simulink model "power_13NodeTestFeedermodel"  (R2021b)
settings: Solver=ode45  StartTime=0.0  StopTime=16  MaxStep=0.04  RelTol=1e-3
PreLoadFcn:
  | power_13NodeTestFeeder_init;
  | Ts=50e-6
values from neighbouring files (symbols this model uses):
  C_dc = 0.008*(n)    (= 1.6)    [VSM.m]
  C_f = n*300*10^-6    (= 0.06)    [VSM.m]
  D_p = (1/(m_p*w_b))    (= 844.343197019)    [VSM.m]
  i_ll = -1.15*(S_b/Vdc_n)-i_loss_dc    [VSM.m]
  i_ul = 1.15*(S_b/Vdc_n)+i_loss_dc    [VSM.m]
  J = D_p*tau_f    (= 16.8868639404)    [VSM.m]
  k_dc = eta_1/(Vdc_n*m_p)    [VSM.m]
  K_p = (1/Vdc_n)    [VSM.m]
  K_r = 1/R_dc    [VSM.m]
  Kff_i = 1    [VSM.m]
  Kff_v = 1    [VSM.m]
  Ki_i = (1/n)*1.19    (= 0.00595)    [VSM.m]
  Ki_v = (n)*1.161022    (= 232.2044)    [VSM.m]
  ki_v_ac = 4*5.2500e-04    (= 0.0021)    [VSM.m]
  Kp_i = 0.738891    [VSM.m]
  Kp_v = 0.52    [VSM.m]
  kp_v_ac = 0.001    [VSM.m]
  L_f = (1/n)*200*10^-6    (= 1e-06)    [VSM.m]
  n = 200    [VSM.m]
  ps = base/3    (= 0.75)    [VSM.m]
  R_dc = (Vdc_n/(0.05*(S_b)/Vdc_n))    [VSM.m]
  R_f = 0.001/n    (= 5e-06)    [VSM.m]
  S_b = 1*(10^6)    (= 1000000)    [VSM.m]
  T_en = T_load-0.5    (= 24.5)    [VSM.m]
  tau_dc = 0.05    [VSM.m]
  V_m = sqrt(2/3)*V1_rms    [VSM.m]
  Vdc_n = 3*V_m    [VSM.m]
  w_b = 2*pi*f_b    (= 376.991118431)    [VSM.m]
  w_f = 2*pi*60    (= 376.991118431)    [VSM.m]
undefined symbols (not defined in the file or in its folder): C_601, C_602, C_603, C_604, C_605, C_606, C_607, ft2km, i_dc, L_601, L_602, L_603, L_604, L_605, L_606, L_607, R_601, R_602, R_603, R_604, R_605, R_606, R_607
libraries: spsSeriesRLCBranchLib x16, spsabctodq0Lib x16, spsVoltageMeasurementLib x14, spsCurrentMeasurementLib x12, spsGroundLib x12, spsLoadFlowBusLib x12, spsPiSectionLineLib x9, spsThreePhaseSeriesRLCLoadLib x7, spsMultimeterLib x6, spsPowerPhasorLib x6, spsThreePhaseVIMeasurementLib x5, spsSeriesRLCLoadLib x5
(part 1 of 2)
settings Model: Creator=The MathWorks, Inc.  LastModifiedBy=aes21009
settings SolverCC: ZeroCrossAlgorithm=Adaptive  AlgebraicLoopSolver=TrustRegion
settings DataIOCC: ExternalInput=getinputstruct(op_IEEE_13_node_5)  InitialState=getstatestruct(op_IEEE_13_node_5)  LimitDataPoints=on  SaveFormat=Array  ReturnWorkspaceOutputs=off
settings OptimizationCC: LifeSpan=inf
settings DebuggingCC: AlgebraicLoopMsg=none  IgnoredZcDiagnostic=none  FcnCallInpInsideContextMsg=warning  UnconnectedInputMsg=none  UnconnectedOutputMsg=none  UnconnectedLineMsg=none  StateNameClashWarn=warning  SFUnexpectedBacktrackingDiag=warning  SFNoUnconditionalDefaultTransitionDiag=warning  SFExecutionAtInitializationDiag=none  SFMachineParentedDataDiag=warning
settings ModelReferenceCC: PropagateSignalLabelsOutOfModel=off
settings SFSimCC: CustomCodeUndefinedFunction=UseInterfaceOnly
settings CodeAppCC: StateflowObjectComments=on
settings SimscapeCC: SimscapeNormalizeSystem=off

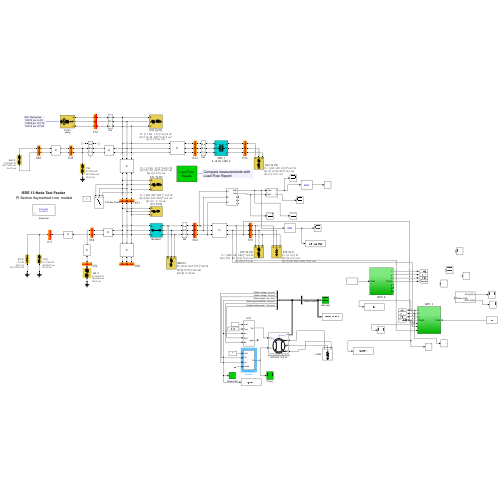
[thumbnail: Simulink's stored preview of the top-level diagram]
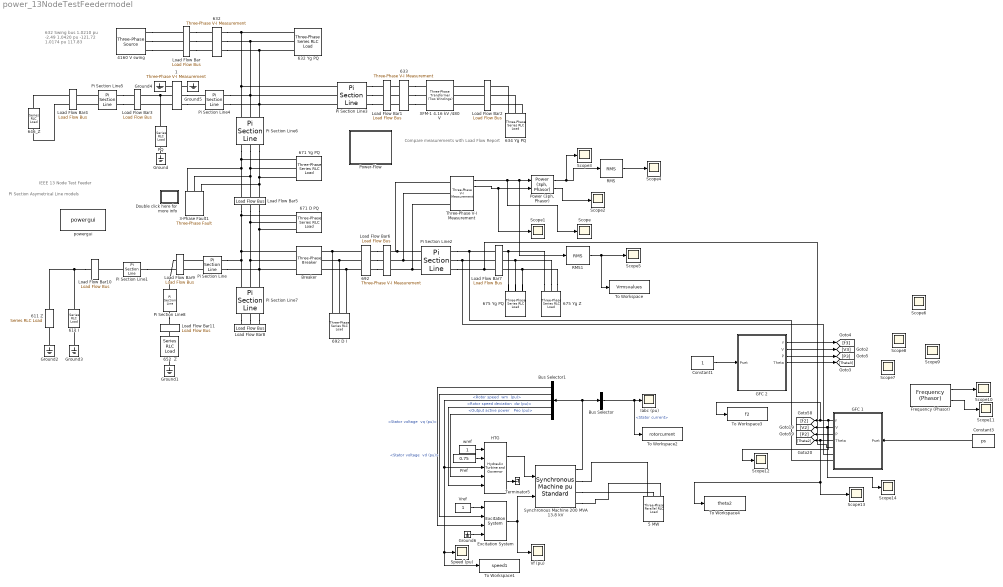
== system power_13NodeTestFeedermodel ==
  note: Compare measurements with
      | Load Flow Report
  note: 632 Swing bus
      | 1.0210 pu -2.49
      | 1.0420 pu -121.72
      | 1.0174 pu 117.83
  note: PI Section Asymetrical Line models
  note: IEEE 13 Node Test Feeder
  " 634 Yg PQ " : spsThreePhaseSeriesRLCLoadLib/Three-Phase Series RLC Load  LConnTagsString=A|B|C  Configuration=Y (grounded)  NominalVoltage=120e3  Vabc=[ 0.993926 1.02168 0.995885]*277.128  Vabcp=[1e3 1e3 1e3]  NominalFrequency=60  UnbalancedPower=on  ActivePower=1e+006  InductivePower=0  CapacitivePower=0  Pabc=[160 120 120]*1e3  QLabc=[110 90 90]*1e3  QCabc=[0 0 0]  Pabcp=[10e3 9e3 11e3]  QLabcp=[100 90 110]  QCabcp=[100 90 110]  Measurements=None  LoadType=constant PQ
      settings: AttributesFormatString=|
      | P= %<Pabc> W
      | Ql=%<QLabc> var
      | Qc=%<QCabc> var
  " Iabc (pu)" : Scope
  " Speed (pu)" : Scope
  1 : spsThreePhaseVIMeasurementLib/Three-Phase V-I Measurement  VoltageMeasurement=phase-to-ground  SetLabelV=on  LabelV=Vabc_645  Vpu=off  VpuLL=off  CurrentMeasurement=yes  SetLabelI=on  LabelI=Iabc_645  Ipu=off  Pbase=100e6  Vbase=4160  OutputType=Complex  PhasorSimulation=off  PSBequivalent=0
  3-Phase Fault1 : spsThreePhaseFaultLib/Three-Phase Fault  InitialStates=0  FaultA=on  FaultB=on  FaultC=on  GroundFault=on  SwitchTimes=[10.1 10.2]  External=off  SwitchStatus=NaN  FaultResistance=1e-3  GroundResistance=1e-3  SnubberResistance=inf  SnubberCapacitance=inf  Measurements=None
  4160 V swing : spsThreePhaseSourceLib/Three-Phase Source  InternalConnection=Yg  VoltagePhases=on  Voltage=120e3  PhaseAngle=0  Voltage_phases=[ 1.021 1.042 1.0174]*2401.78  PhaseAngles_phases=[ -2.49006 -121.72 117.83]  Frequency=60  NonIdealSource=on  SpecifyImpedance=off  Resistance=1e-5  Inductance=0  ShortCircuitLevel=100e6  BaseVoltage=120e3  XRratio=10  BusType=swing  Pref=0  Qref=0  Prefabc=[0 0 0]  Qrefabc=[0 0 0]  Qmin="[-inf  -inf -inf]"  Qmax="[inf  inf inf]"
  5 MW : spsThreePhaseParallelRLCLoadLib/Three-Phase Parallel RLC Load  LConnTagsString=A|B|C  Configuration=Y (grounded)  NominalVoltage=4160  Vabc=[1e3 1e3 1e3]  Vabcp=[1e3 1e3 1e3]  NominalFrequency=60  UnbalancedPower=off  ActivePower=50000  InductivePower=0  CapacitivePower=0  Pabc=[10e3 9e3 11e3]  QLabc=[100 90 110]  QCabc=[100 90 110]  Pabcp=[10e3 9e3 11e3]  QLabcp=[100 90 110]  QCabcp=[100 90 110]  Measurements=None  LoadType=constant Z
  611 I : spsSeriesRLCLoadLib/Series RLC Load  LConnTagsString=a  RConnTagsString=__new0  NominalVoltage=0.986755*2401.78  NominalFrequency=60  ActivePower=170e3  InductivePower=80e3  CapacitivePower=0  Setx0=off  InitialVoltage=0  SetiL0=off  InitialCurrent=0  Measurements=Branch voltage and current  LoadType=constant I
      settings: AttributesFormatString=|
      | P=%<ActivePower> W
      | Ql=%<InductivePower> var
      | Qc=%<CapacitivePower> var
  611 Z : spsSeriesRLCLoadLib/Series RLC Load  LConnTagsString=a  RConnTagsString=__new0  NominalVoltage=4160/sqrt(3)  NominalFrequency=60  ActivePower=0  InductivePower=0  CapacitivePower=100e3  Setx0=off  InitialVoltage=0  SetiL0=off  InitialCurrent=0  Measurements=None  LoadType=constant Z
      settings: AttributesFormatString=|
      | P=%<ActivePower> W
      | Ql=%<InductivePower> var
      | Qc=%<CapacitivePower> var
  632 : spsThreePhaseVIMeasurementLib/Three-Phase V-I Measurement  VoltageMeasurement=phase-to-ground  SetLabelV=on  LabelV=Vabc_632  Vpu=off  VpuLL=off  CurrentMeasurement=yes  SetLabelI=on  LabelI=Iabc_632  Ipu=off  Pbase=100e6  Vbase=4160  OutputType=Complex  PhasorSimulation=off  PSBequivalent=0
  632 Yg PQ : spsThreePhaseSeriesRLCLoadLib/Three-Phase Series RLC Load  LConnTagsString=A|B|C  Configuration=Y (grounded)  NominalVoltage=120e3  Vabc=[ 1.021 1.042 1.0174]*2401.78  Vabcp=[1e3 1e3 1e3]  NominalFrequency=60  UnbalancedPower=on  ActivePower=1e+006  InductivePower=0  CapacitivePower=0  Pabc="[17 66  117]*1e3/2"  QLabc="[10 38  68]*1e3/2"  QCabc=[0 0 0]  Pabcp=[10e3 9e3 11e3]  QLabcp=[100 90 110]  QCabcp=[100 90 110]  Measurements=None  LoadType=constant PQ
      settings: AttributesFormatString=|
      | P= %<Pabc> W
      | Ql=%<QLabc> var
      | Qc=%<QCabc> var
  633 : spsThreePhaseVIMeasurementLib/Three-Phase V-I Measurement  VoltageMeasurement=phase-to-ground  SetLabelV=on  LabelV=Vabc_633  Vpu=off  VpuLL=off  CurrentMeasurement=yes  SetLabelI=on  LabelI=Iabc_633  Ipu=off  Pbase=100e6  Vbase=4160  OutputType=Complex  PhasorSimulation=off  PSBequivalent=0
  646_Z : spsSeriesRLCLoadLib/Series RLC Load  LConnTagsString=a  RConnTagsString=__new0  NominalVoltage=4160  NominalFrequency=60  ActivePower=230e3  InductivePower=132e3  CapacitivePower=0  Setx0=off  InitialVoltage=0  SetiL0=off  InitialCurrent=0  Measurements=None  LoadType=constant Z
      settings: AttributesFormatString=|
      | P=%<ActivePower> W
      | Ql=%<InductivePower> var
      | Qc=%<CapacitivePower> var
  "652  Z " : spsSeriesRLCLoadLib/Series RLC Load  LConnTagsString=a  RConnTagsString=__new0  NominalVoltage=4160/sqrt(3)  NominalFrequency=60  ActivePower=128e3  InductivePower=86e3  CapacitivePower=0  Setx0=off  InitialVoltage=0  SetiL0=off  InitialCurrent=0  Measurements=None  LoadType=constant Z
      settings: AttributesFormatString=|
      | P=%<ActivePower> W
      | Ql=%<InductivePower> var
      | Qc=%<CapacitivePower> var
  671 D PQ : spsThreePhaseSeriesRLCLoadLib/Three-Phase Series RLC Load  LConnTagsString=A|B|C  Configuration=Delta  NominalVoltage=120e3  Vabc="[1  1  1]*120e3/sqrt(3)"  Vabcp=[ 1.7426 1.77325 1.71534]*2401.78  NominalFrequency=60  UnbalancedPower=on  ActivePower=1e+006  InductivePower=0  CapacitivePower=0  Pabc="[17 66  117]*1e3/2"  QLabc="[10 38  68]*1e3/2"  QCabc=[0 0 0]  Pabcp=[385 385 385 ]*1e3  QLabcp=[220 220 220]*1e3  QCabcp="[0  0  0]"  Measurements=Branch voltages and currents  LoadType=constant PQ
      settings: AttributesFormatString=|
      | P= %<Pabcp> W
      | Ql=%<QLabcp> var
      | Qc=%<QCabcp> var
  671 Yg PQ : spsThreePhaseSeriesRLCLoadLib/Three-Phase Series RLC Load  LConnTagsString=A|B|C  Configuration=Y (grounded)  NominalVoltage=120e3  Vabc=[ 0.990007 1.05293 0.977696]*2401.78  Vabcp=[1e3 1e3 1e3]  NominalFrequency=60  UnbalancedPower=on  ActivePower=1e+006  InductivePower=0  CapacitivePower=0  Pabc="[17 66  117]*1e3/2"  QLabc="[10 38  68]*1e3/2"  QCabc=[0 0 0]  Pabcp=[10e3 9e3 11e3]  QLabcp=[100 90 110]  QCabcp=[100 90 110]  Measurements=None  LoadType=constant PQ
      settings: AttributesFormatString=|
      | P= %<Pabc> W
      | Ql=%<QLabc> var
      | Qc=%<QCabc> var
  675 Yg PQ : spsThreePhaseSeriesRLCLoadLib/Three-Phase Series RLC Load  LConnTagsString=A|B|C  Configuration=Y (grounded)  NominalVoltage=120e3  Vabc=[ 0.983621 1.05532 0.975578]*2401.78  Vabcp=[1e3 1e3 1e3]  NominalFrequency=60  UnbalancedPower=on  ActivePower=1e+006  InductivePower=0  CapacitivePower=0  Pabc="[485  68  290]*1e3"  QLabc="[190  60  212]*1e3"  QCabc=[0 0 0]  Pabcp=[10e3 9e3 11e3]  QLabcp=[100 90 110]  QCabcp=[100 90 110]  Measurements=Branch voltages and currents  LoadType=constant PQ
      settings: AttributesFormatString=|
      | P= %<Pabc> W
      | Ql=%<QLabc> var
      | Qc=%<QCabc> var
  675 Yg Z : spsThreePhaseSeriesRLCLoadLib/Three-Phase Series RLC Load  LConnTagsString=A|B|C  Configuration=Y (grounded)  NominalVoltage=120e3  Vabc="[1  1  1]*4160/sqrt(3)"  Vabcp=[1e3 1e3 1e3]  NominalFrequency=60  UnbalancedPower=on  ActivePower=1e+006  InductivePower=0  CapacitivePower=0  Pabc=[0 0 0]  QLabc=[0 0 0]  QCabc=[200 200 200]*1e3  Pabcp=[10e3 9e3 11e3]  QLabcp=[100 90 110]  QCabcp=[100 90 110]  Measurements=None  LoadType=constant Z
      settings: AttributesFormatString=|
      | P= %<Pabc> W
      | Ql=%<QLabc> var
      | Qc=%<QCabc> var
  692 : spsThreePhaseVIMeasurementLib/Three-Phase V-I Measurement  VoltageMeasurement=phase-to-ground  SetLabelV=on  LabelV=Vabc_692  Vpu=off  VpuLL=off  CurrentMeasurement=yes  SetLabelI=on  LabelI=Iabc_692  Ipu=off  Pbase=100e6  Vbase=4160  OutputType=Complex  PhasorSimulation=off  PSBequivalent=0
  692 D I : spsThreePhaseSeriesRLCLoadLib/Three-Phase Series RLC Load  LConnTagsString=A|B|C  Configuration=Delta  NominalVoltage=120e3  Vabc="[1  1  1]*120e3/sqrt(3)"  Vabcp=[ 1.73731 1.75253 1.72367]*2401.78  NominalFrequency=60  UnbalancedPower=on  ActivePower=1e+006  InductivePower=0  CapacitivePower=0  Pabc="[17 66  117]*1e3/2"  QLabc="[10 38  68]*1e3/2"  QCabc=[0 0 0]  Pabcp=[1e-6 1e-6 170 ]*1e3  QLabcp=[0 0 151]*1e3  QCabcp="[0  0  0]"  Measurements=Branch voltages and currents  LoadType=constant I
      settings: AttributesFormatString=|
      | P= %<Pabcp> W
      | Ql=%<QLabcp> var
      | Qc=%<QCabcp> var
  Breaker : spsThreePhaseBreakerLib/Three-Phase Breaker  InitialState=closed  SwitchA=on  SwitchB=on  SwitchC=on  SwitchTimes=[ 12 ]  External=off  BreakerResistance=0.0001  SnubberResistance=inf  SnubberCapacitance=0  Measurements=Breaker voltages and currents
  Bus Selector : BusSelector  OutputSignals=Stator current
  Bus Selector1 : BusSelector  OutputSignals="dq0 components.Stator voltage  vq (pu),dq0 components.Stator voltage  vd (pu),Mechanical.Rotor speed  wm  (pu),Mechanical.Rotor speed deviation  dw (pu),Output active power   Peo (pu)"
  Constant1 : Constant
  Constant3 : Constant  Value=ps
  Double click here for more info : Subsystem
      settings: OpenFcn=showdemo(bdroot(gcb))
      mask Display: disp('?')
  Excitation System : spsExcitationSystemLib/Excitation System  tr=20e-3  reg=[ 300, 0.001 ]  exc=[ 1, 0 ]  tgr=[ 0, 0 ]  damp=[ 0.001, 0.1 ]  sat=[ 0, 0 ]  lim=[ -11.5, 11.5, 0 ]  v0=[1,1.29071]
      settings: SourceProductBaseCode=PS
  Frequency (Phasor) : spsFrequencyPhasorLib/Frequency (Phasor)  Fn=60  T=0.1
      settings: SourceProductBaseCode=PS
  GFC 1 : Subsystem
  GFC 2 : Subsystem
  Ground{,1..5} (6 alike) : spsGroundLib/Ground  LConnTagsString=a
  Ground6 : Ground
  HTG : spsHydraulicTurbineandGovernorLib/Hydraulic Turbine and Governor  sm="[ 10/3  0.07 ]"  gate="[  0.01  0.97518  -0.1  0.1 ]"  reg="[  0.05  1.163  0.105  0  0.01  ]"  hyd="[  0  2.67  ]"  dref=0  po=0.751606
      settings: SourceProductBaseCode=PS
  Load Flow Bar : spsLoadFlowBusLib/Load Flow Bus  LConnTagsString=a|b|c  RConnTagsString=a|b|c  Phases=ABC  Connectors=on both sides  ID=632  Vbase=4160/sqrt(3)  Vref="[ 1.0210  1.0420  1.0174]"  Vangle="[ -2.49  -121.72  117.83]"  VLF=1.021  VLFb=1.042  VLFc=1.017  angleLF=-2.49  angleLFb=-121.7  angleLFc=117.8
      settings: AttributesFormatString=%<ID>  SourceProductBaseCode=PS
  Load Flow Bar1 : spsLoadFlowBusLib/Load Flow Bus  LConnTagsString=a|b|c  RConnTagsString=a|b|c  Phases=ABC  Connectors=on both sides  ID=633  Vbase=4160/sqrt(3)  Vref=[1.0 1.0 1.0]  Vangle=[0 -120 120]  VLF=1.018  VLFb=1.04  VLFc=1.015  angleLF=-2.555  angleLFb=-121.8  angleLFc=117.8
      settings: AttributesFormatString=%<ID>  SourceProductBaseCode=PS
  Load Flow Bar10 : spsLoadFlowBusLib/Load Flow Bus  LConnTagsString=a  RConnTagsString=a  Phases=C  Connectors=on both sides  ID=611  Vbase=4160/sqrt(3)  Vref=1.0  Vangle=0  VLF=NaN  VLFb=NaN  VLFc=0.9737  angleLF=NaN  angleLFb=NaN  angleLFc=115.8
      settings: AttributesFormatString=%<ID>  SourceProductBaseCode=PS
  Load Flow Bar11 : spsLoadFlowBusLib/Load Flow Bus  LConnTagsString=a  RConnTagsString=a  Phases=A  Connectors=on both sides  ID=652  Vbase=4160/sqrt(3)  Vref=1.0  Vangle=0  VLF=0.9825  VLFb=NaN  VLFc=NaN  angleLF=-5.246  angleLFb=NaN  angleLFc=NaN
      settings: AttributesFormatString=%<ID>  SourceProductBaseCode=PS
  Load Flow Bar2 : spsLoadFlowBusLib/Load Flow Bus  LConnTagsString=a|b|c  RConnTagsString=a|b|c  Phases=ABC  Connectors=on both sides  ID=634  Vbase=480/sqrt(3)  Vref=[1.0 1.0 1.0]  Vangle=[0 -120 120]  VLF=0.9939  VLFb=1.022  VLFc=0.9959  angleLF=-3.232  angleLFb=-122.2  angleLFc=117.3
      settings: AttributesFormatString=%<ID>  SourceProductBaseCode=PS
  Load Flow Bar3 : spsLoadFlowBusLib/Load Flow Bus  LConnTagsString=a|b  RConnTagsString=a|b  Phases=BC  Connectors=on both sides  ID=645  Vbase=4160/sqrt(3)  Vref=[1.0 1.0 ]  Vangle=[0 0]  VLF=NaN  VLFb=1.033  VLFc=1.015  angleLF=NaN  angleLFb=-121.9  angleLFc=117.9
      settings: AttributesFormatString=%<ID>  SourceProductBaseCode=PS
  Load Flow Bar4 : spsLoadFlowBusLib/Load Flow Bus  LConnTagsString=a|b  RConnTagsString=a|b  Phases=BC  Connectors=on both sides  ID=646  Vbase=4160/sqrt(3)  Vref=[1.0 1.0 ]  Vangle=[0 0]  VLF=NaN  VLFb=1.031  VLFc=1.013  angleLF=NaN  angleLFb=-122  angleLFc=117.9
      settings: AttributesFormatString=%<ID>  SourceProductBaseCode=PS
  Load Flow Bar5 : spsLoadFlowBusLib/Load Flow Bus  LConnTagsString=a|b|c  RConnTagsString=a|b|c  Phases=ABC  Connectors=on both sides  ID=671  Vbase=4160/sqrt(3)  Vref=[1.0 1.0 1.0]  Vangle=[0 -120 120]  VLF=0.99  VLFb=1.053  VLFc=0.9777  angleLF=-5.298  angleLFb=-122.3  angleLFc=116
      settings: AttributesFormatString=%<ID>  SourceProductBaseCode=PS
  Load Flow Bar6 : spsLoadFlowBusLib/Load Flow Bus  LConnTagsString=a|b|c  RConnTagsString=a|b|c  Phases=ABC  Connectors=on both sides  ID=692  Vbase=4160/sqrt(3)  Vref=[1.0 1.0 1.0]  Vangle=[0 -120 120]  VLF=0.99  VLFb=1.053  VLFc=0.9777  angleLF=-5.298  angleLFb=-122.3  angleLFc=116
      settings: AttributesFormatString=%<ID>  SourceProductBaseCode=PS
  Load Flow Bar7 : spsLoadFlowBusLib/Load Flow Bus  LConnTagsString=a|b|c  RConnTagsString=a|b|c  Phases=ABC  Connectors=on both sides  ID=675  Vbase=4160/sqrt(3)  Vref=[1.0 1.0 1.0]  Vangle=[0 -120 120]  VLF=0.9836  VLFb=1.055  VLFc=0.9756  angleLF=-5.544  angleLFb=-122.5  angleLFc=116
      settings: AttributesFormatString=%<ID>  SourceProductBaseCode=PS
  Load Flow Bar8 : spsLoadFlowBusLib/Load Flow Bus  LConnTagsString=a|b|c  Phases=ABC  Connectors=on one side  ID=680  Vbase=4160/sqrt(3)  Vref=[1.0 1.0 1.0]  Vangle=[0 -120 120]  VLF=0.99  VLFb=1.053  VLFc=0.9777  angleLF=-5.298  angleLFb=-122.3  angleLFc=116
      settings: AttributesFormatString=%<ID>  SourceProductBaseCode=PS
  Load Flow Bar9 : spsLoadFlowBusLib/Load Flow Bus  LConnTagsString=a|b  RConnTagsString=a|b  Phases=AC  Connectors=on both sides  ID=684  Vbase=4160/sqrt(3)  Vref=[1.0 1.0 ]  Vangle=[0 -120 ]  VLF=0.9881  VLFb=NaN  VLFc=0.9757  angleLF=-5.321  angleLFb=NaN  angleLFc=115.9
      settings: AttributesFormatString=%<ID>  SourceProductBaseCode=PS
  PQ : spsSeriesRLCLoadLib/Series RLC Load  LConnTagsString=a  RConnTagsString=__new0  NominalVoltage=1.03283*2401.78  NominalFrequency=60  ActivePower=170e3  InductivePower=125e3  CapacitivePower=0  Setx0=off  InitialVoltage=0  SetiL0=off  InitialCurrent=0  Measurements=None  LoadType=constant PQ
      settings: AttributesFormatString=|
      | P=%<ActivePower> W
      | Ql=%<InductivePower> var
      | Qc=%<CapacitivePower> var
  Pi Section Line : spsPiSectionLineLib/Pi Section Line  LConnTagsString=1|i2  RConnTagsString=1|o2  Phases=2  PiSections=1  Length=300*ft2km  Frequency=60  Resistance=R_604([1 3],[1 3])  Inductance=L_604([1 3],[1 3])  Capacitance=C_604([1 3],[1 3])  Measurements=None  Measurements2=None
      settings: SourceProductBaseCode=PS
  Pi Section Line1 : spsPiSectionLineLib/Pi Section Line  LConnTagsString=1  RConnTagsString=1  Phases=1  PiSections=1  Length=300*ft2km  Frequency=60  Resistance=R_605(3,3)  Inductance=L_605(3,3)  Capacitance=C_605(3,3)  Measurements=None  Measurements2=None
      settings: SourceProductBaseCode=PS
  Pi Section Line2 : spsPiSectionLineLib/Pi Section Line  LConnTagsString=1|i2|i3  RConnTagsString=1|o2|o3  Phases=3  PiSections=1  Length=500*ft2km  Frequency=60  Resistance=R_606  Inductance=L_606  Capacitance=C_606  Measurements=None  Measurements2=None
      settings: SourceProductBaseCode=PS
  Pi Section Line3 : spsPiSectionLineLib/Pi Section Line  LConnTagsString=1|i2|i3  RConnTagsString=1|o2|o3  Phases=3  PiSections=1  Length=500*ft2km  Frequency=60  Resistance=R_602  Inductance=L_602  Capacitance=C_602  Measurements=None  Measurements2=None
      settings: SourceProductBaseCode=PS
  Pi Section Line4 : spsPiSectionLineLib/Pi Section Line  LConnTagsString=1|i2  RConnTagsString=1|o2  Phases=2  PiSections=1  Length=500*ft2km  Frequency=60  Resistance=R_603(2:3,2:3)  Inductance=L_603(2:3,2:3)  Capacitance=C_603(2:3,2:3)  Measurements=None  Measurements2=None
      settings: SourceProductBaseCode=PS
  Pi Section Line5 : spsPiSectionLineLib/Pi Section Line  LConnTagsString=1|i2  RConnTagsString=1|o2  Phases=2  PiSections=1  Length=300*ft2km  Frequency=60  Resistance=R_603(2:3,2:3)  Inductance=L_603(2:3,2:3)  Capacitance=C_603(2:3,2:3)  Measurements=None  Measurements2=None
      settings: SourceProductBaseCode=PS
  Pi Section Line6 : spsPiSectionLineLib/Pi Section Line  LConnTagsString=1|i2|i3  RConnTagsString=1|o2|o3  Phases=3  PiSections=1  Length=2000*ft2km  Frequency=60  Resistance=R_601  Inductance=L_601  Capacitance=C_601  Measurements=None  Measurements2=None
      settings: SourceProductBaseCode=PS
  Pi Section Line7 : spsPiSectionLineLib/Pi Section Line  LConnTagsString=1|i2|i3  RConnTagsString=1|o2|o3  Phases=3  PiSections=1  Length=1000*ft2km  Frequency=60  Resistance=R_601  Inductance=L_601  Capacitance=C_601  Measurements=None  Measurements2=None
      settings: SourceProductBaseCode=PS
  Pi Section Line8 : spsPiSectionLineLib/Pi Section Line  LConnTagsString=1  RConnTagsString=1  Phases=1  PiSections=1  Length=800*ft2km  Frequency=60  Resistance=R_607(1,1)  Inductance=L_607(1,1)  Capacitance=C_607(1,1)  Measurements=None  Measurements2=None
      settings: SourceProductBaseCode=PS
  "Power (3ph, Phasor)" : spsPower3phPhasorLib/Power (3ph, Phasor)
      settings: SourceProductBaseCode=PS
  Power-Flow : Subsystem
      mask Display: disp('Load Flow\nResults')
  Pref : Constant  Value=0.75
  RMS : spsRMSLib/RMS  TrueRMS=on  Freq=60  RMSInit=120  Ts=0
  RMS1 : spsRMSLib/RMS  TrueRMS=on  Freq=60  RMSInit=120  Ts=0
  Scope{,1..14} (15 alike) : Scope
  Synchronous Machine 200 MVA 13.8 kV : spsSynchronousMachinepuStandardLib/Synchronous Machine pu Standard  PresetModel=No  MechanicalLoad=Mechanical power Pm  ShowDetailedParameters=on  RotorType=Salient-pole  Units=per unit standard parameters  MeasurementBus=off  NominalParameters="[1E6  4160  60 ]"  Reactances1=[ 31 32 33 34 35 36 37 ]  Reactances2=[ 1.305, 0.296, 0.252, 0.474, 0.243, 0.18 ]  dAxisTimeConstants=Short-circuit  qAxisTimeConstants=Open-circuit  TimeConstants1=[]  TimeConstants2=[]  TimeConstants3=[]  TimeConstants4=[]  TimeConstants5=[ 1.01, 0.053, 0.1 ]  TimeConstants6=[]  TimeConstants7=[]  TimeConstants8=[]  StatorResistance=2.8544e-3  Mechanical=[ 3.2 0 2]  PolePairs=2  InitialConditions=[0 -94.2826 0.750185 0.750185 0.750185 -24.943 -144.943 95.057 1.29071]  SetSaturation=off  Saturation=[0.6404,0.7127,0.8441,0.9214,0.9956,1.082,1.19,1.316,1.457;0.7,0.7698,0.8872,0.9466,0.9969,1.046,1.1,1.151,1.201]  LoadFlowParameters=[1 150000000 0 0]  TsPowergui=0  TsBlock=-1  IterativeModel=Trapezoidal non iterative  IterativeDiscreteModel=Trapezoidal non iterative  BusType=PV  Pref=150000000  Qref=0  Qmin=-Inf  Qmax=Inf  PLF=0  QLF=0
      settings: SourceProductBaseCode=PS
  Terminator5 : Terminator
  Three-Phase V-I Measurement : spsThreePhaseVIMeasurementLib/Three-Phase V-I Measurement  VoltageMeasurement=phase-to-ground  SetLabelV=off  LabelV=Vabc  Vpu=off  VpuLL=off  CurrentMeasurement=yes  SetLabelI=off  LabelI=Iabc  Ipu=off  Pbase=100e6  Vbase=500e3  OutputType=Complex  PhasorSimulation=off  PSBequivalent=0
  To Workspace : ToWorkspace  VariableName=Vrmsvalues  SampleTime=-1
  To Workspace1 : ToWorkspace  VariableName=speed1  SampleTime=-1
  To Workspace2 : ToWorkspace  VariableName=rotorcurrent  SaveFormat=Timeseries  SampleTime=-1
  To Workspace3 : ToWorkspace  VariableName=f2  SampleTime=-1
  To Workspace4 : ToWorkspace  VariableName=theta2  SampleTime=-1
  Vf (pu) : Scope
  Vref : Constant
  XFM-1 4.16 kV /480 V : spsThreePhaseTransformerTwoWindingsLib/Three-Phase Transformer (Two Windings)  Winding1Connection=Yg  Winding2Connection=Yg  CoreType=Three single-phase transformers  SetSaturation=off  Hysteresis=off  DataFile='hysteresis'  SetInitialFlux=off  Measurements=None  UNITS=pu  NominalPower=[ 500e3 , 60 ]  Winding1=[4160 0.011 0.02]  Winding2=[480 0 0]  Rm=500  Lm=500  L0=0.5  Saturation=[0 0;0.0024 1.2;1 1.52]  InitialFluxes=[0.8 -0.8 0.7]  BreakLoop=off  DiscreteSolver=Trapezoidal iterative  DataType=off  TransfoNumber=1
  powergui : spspowerguiLib/powergui  Priority=1  SimulationMode=Discrete  SampleTime=0.00001  frequency=60  Iterations=50  frequencyindice=60  Pbase=100e3  ErrMax=0.0001  UnitsV=kV  UnitsW=kW  buscounter=0  FunctionMessages=off  echomessages=off  EnableUseOfTLC=off  CurrentSourceSwitches=off  DisableSnubberDevices=off  DisableRonSwitches=off  DisableVfSwitches=off  DisplayEquations=off  AutomaticDiscreteSolvers=off  SolverType=Tustin/Backward Euler (TBE)  Interpol=off  ExternalGateDelay=off  methode=off  Ts=0  x0status=blocks  SPID=off  SwTol=0  HookPort=off  NonlinearTolerance=1e-4  nMaxIteration=100  ContinueOnMaxIteration=off  RestoreLinks=warning  ResistiveCurrentMeasurement=off  Frange=[0:2:500]  Ylog=off  Xlog=on  ShowGrid=off  save=off  variable=ZData  structure=0  ZoomFFT=on  StartTime=0.0  cycles=1  DisplayStyle=1  fundamental=60  FreqAxis=off  MaxFrequency=1000  frequencyindicesteady=1  RmsSteady=1  display=off
  wref : Constant
  wires:
  Three-Phase V-I Measurement/1 -> Scope/1, RMS1/1, "Power (3ph, Phasor)"/1
  Three-Phase V-I Measurement/2 -> Scope1/1, "Power (3ph, Phasor)"/2
  "Power (3ph, Phasor)"/1 -> Scope3/1, RMS/1
  "Power (3ph, Phasor)"/2 -> Scope2/1
  RMS/1 -> Scope4/1
  RMS1/1 -> To Workspace/1, Scope5/1
  Bus Selector1/5 -> HTG/4  "<Output active power   Peo (pu)>"
  Excitation System/1 -> Vf (pu)/1, Synchronous Machine 200 MVA 13.8 kV/2
  Bus Selector1/2 -> Excitation System/2  "<Stator voltage  vd (pu)>"
  Pref/1 -> HTG/2
  Bus Selector1/1 -> Excitation System/3  "<Stator voltage  vq (pu)>"
  HTG/1 -> Synchronous Machine 200 MVA 13.8 kV/1
  Bus Selector1/3 -> HTG/3, To Workspace1/1, " Speed (pu)"/1  "<Rotor speed  wm  (pu)>"
  Bus Selector/1 -> To Workspace2/1, " Iabc (pu)"/1  "<Stator current>"
  Bus Selector1/4 -> HTG/5  "<Rotor speed deviation  dw (pu)>"
  Synchronous Machine 200 MVA 13.8 kV/1 -> Bus Selector/1, Bus Selector1/1
  Ground6/1 -> Excitation System/4
  wref/1 -> HTG/1
  HTG/2 -> Terminator5/1
  Vref/1 -> Excitation System/1
  GFC 1/1(f) -> Scope12/1, To Workspace3/1, [f2]
  GFC 1/2(V) -> Scope14/1, [V2]
  GFC 1/3(P) -> [P2]
  GFC 2/2(V) -> [V3]
  Constant1/1 -> GFC 2/1(Pset)
  Constant3/1 -> GFC 1/1(Pset)
  GFC 2/1(f) -> [f3]
  GFC 2/3(P) -> [P3]
  GFC 2/4(Theta) -> [Theta3]
  Frequency (Phasor)/1 -> Scope10/1
  Frequency (Phasor)/2 -> Scope11/1
  GFC 1/4(Theta) -> [Theta2], To Workspace4/1, Scope13/1
  connections:
  632/RConn2 -- 632 Yg PQ/LConn2 -- Pi Section Line4/RConn1 -- Pi Section Line6/LConn2 -- Pi Section Line3/LConn2
  675 Yg Z/LConn1 -- Load Flow Bar7/LConn1 -- 675 Yg PQ/LConn1
  671 D PQ/LConn2 -- Breaker/LConn2 -- Pi Section Line7/LConn2 -- Load Flow Bar5/RConn2
  692 D I/LConn3 -- 692/LConn3 -- Breaker/RConn3
  Pi Section Line/RConn1 -- Pi Section Line7/LConn1 -- 671 D PQ/LConn1 -- Load Flow Bar5/RConn1 -- Breaker/LConn1
  Load Flow Bar3/RConn1 -- 1/LConn2 -- PQ/LConn1
  675 Yg Z/LConn3 -- Load Flow Bar7/LConn3 -- 675 Yg PQ/LConn3
  671 Yg PQ/LConn2 -- 3-Phase Fault1/LConn2 -- Load Flow Bar5/LConn2 -- Pi Section Line6/RConn2
  Load Flow Bar10/LConn1 -- 611 Z/LConn1 -- 611 I/LConn1
  671 Yg PQ/LConn3 -- Pi Section Line6/RConn3 -- 3-Phase Fault1/LConn3 -- Load Flow Bar5/LConn3
  Pi Section Line6/LConn1 -- 632 Yg PQ/LConn1 -- 632/RConn1 -- Pi Section Line3/LConn1
  671 D PQ/LConn3 -- Load Flow Bar5/RConn3 -- Pi Section Line7/LConn3 -- Breaker/LConn3 -- Pi Section Line/RConn2
  632/RConn3 -- 632 Yg PQ/LConn3 -- Pi Section Line4/RConn2 -- Pi Section Line6/LConn3 -- Pi Section Line3/LConn3
  Breaker/RConn1 -- 692 D I/LConn1 -- 692/LConn1
  671 Yg PQ/LConn1 -- 3-Phase Fault1/LConn1 -- Load Flow Bar5/LConn1 -- Pi Section Line6/RConn1
  Breaker/RConn2 -- 692 D I/LConn2 -- 692/LConn2
  675 Yg Z/LConn2 -- Load Flow Bar7/LConn2 -- 675 Yg PQ/LConn2
  692/RConn1 -- Load Flow Bar6/RConn1
  1/LConn3 -- Load Flow Bar3/RConn2
  Ground2/LConn1 -- 611 Z/RConn1
  Pi Section Line1/LConn1 -- Load Flow Bar10/RConn1
  692/RConn3 -- Load Flow Bar6/RConn3
  Pi Section Line5/RConn1 -- Load Flow Bar3/LConn1
  Load Flow Bar2/LConn2 -- XFM-1 4.16 kV /480 V/RConn2
  " 634 Yg PQ "/LConn2 -- Load Flow Bar2/RConn2
  4160 V swing/RConn2 -- Load Flow Bar/LConn2
  Pi Section Line7/RConn3 -- Load Flow Bar8/LConn3
  Pi Section Line5/RConn2 -- Load Flow Bar3/LConn2
  633/LConn1 -- Load Flow Bar1/RConn1
  Pi Section Line2/RConn1 -- GFC 1/RConn3 -- Load Flow Bar7/RConn1
  Ground/LConn1 -- PQ/RConn1
  Pi Section Line/LConn1 -- Load Flow Bar9/RConn1
  Pi Section Line7/RConn1 -- Load Flow Bar8/LConn1
  Load Flow Bar4/LConn2 -- 646_Z/RConn1
  1/RConn3 -- Pi Section Line4/LConn2
  Pi Section Line5/LConn1 -- Load Flow Bar4/RConn1
  Pi Section Line7/RConn2 -- Load Flow Bar8/LConn2
  Pi Section Line8/LConn1 -- Load Flow Bar9/LConn1
  692/RConn2 -- Load Flow Bar6/RConn2
  Ground1/LConn1 -- "652  Z "/RConn1
  Pi Section Line2/LConn1 -- Three-Phase V-I Measurement/LConn1 -- Load Flow Bar6/LConn1
  4160 V swing/RConn1 -- Load Flow Bar/LConn1
  Pi Section Line/LConn2 -- Load Flow Bar9/RConn2
  633/RConn3 -- XFM-1 4.16 kV /480 V/LConn3
  Pi Section Line8/RConn1 -- Load Flow Bar11/LConn1
  4160 V swing/RConn3 -- Load Flow Bar/LConn3
  "652  Z "/LConn1 -- Load Flow Bar11/RConn1
  633/RConn2 -- XFM-1 4.16 kV /480 V/LConn2
  1/RConn1 -- Ground5/LConn1
  633/RConn1 -- XFM-1 4.16 kV /480 V/LConn1
  Pi Section Line2/LConn2 -- Three-Phase V-I Measurement/LConn2 -- Load Flow Bar6/LConn2
  Load Flow Bar/RConn2 -- 632/LConn2
  Ground3/LConn1 -- 611 I/RConn1
  Pi Section Line3/RConn1 -- Load Flow Bar1/LConn1
  Load Flow Bar/RConn1 -- 632/LConn1
  Pi Section Line5/LConn2 -- Load Flow Bar4/RConn2
  Pi Section Line3/RConn2 -- Load Flow Bar1/LConn2
  633/LConn3 -- Load Flow Bar1/RConn3
  Load Flow Bar/RConn3 -- 632/LConn3
  Pi Section Line3/RConn3 -- Load Flow Bar1/LConn3
  633/LConn2 -- Load Flow Bar1/RConn2
  Ground4/LConn1 -- 1/LConn1
  Pi Section Line1/RConn1 -- Load Flow Bar9/LConn2
  Load Flow Bar2/LConn1 -- XFM-1 4.16 kV /480 V/RConn1
  " 634 Yg PQ "/LConn1 -- Load Flow Bar2/RConn1
  Pi Section Line2/LConn3 -- Three-Phase V-I Measurement/LConn3 -- Load Flow Bar6/LConn3
  Load Flow Bar2/LConn3 -- XFM-1 4.16 kV /480 V/RConn3
  1/RConn2 -- Pi Section Line4/LConn1
  " 634 Yg PQ "/LConn3 -- Load Flow Bar2/RConn3
  646_Z/LConn1 -- Load Flow Bar4/LConn1
  Pi Section Line2/RConn2 -- GFC 1/RConn2 -- Load Flow Bar7/RConn2
  Synchronous Machine 200 MVA 13.8 kV/RConn3 -- 5 MW/LConn3
  Synchronous Machine 200 MVA 13.8 kV/RConn1 -- 5 MW/LConn1
  Pi Section Line2/RConn3 -- GFC 1/RConn1 -- Load Flow Bar7/RConn3
  Synchronous Machine 200 MVA 13.8 kV/RConn2 -- 5 MW/LConn2

== system power_13NodeTestFeedermodel/Double click here for more info ==

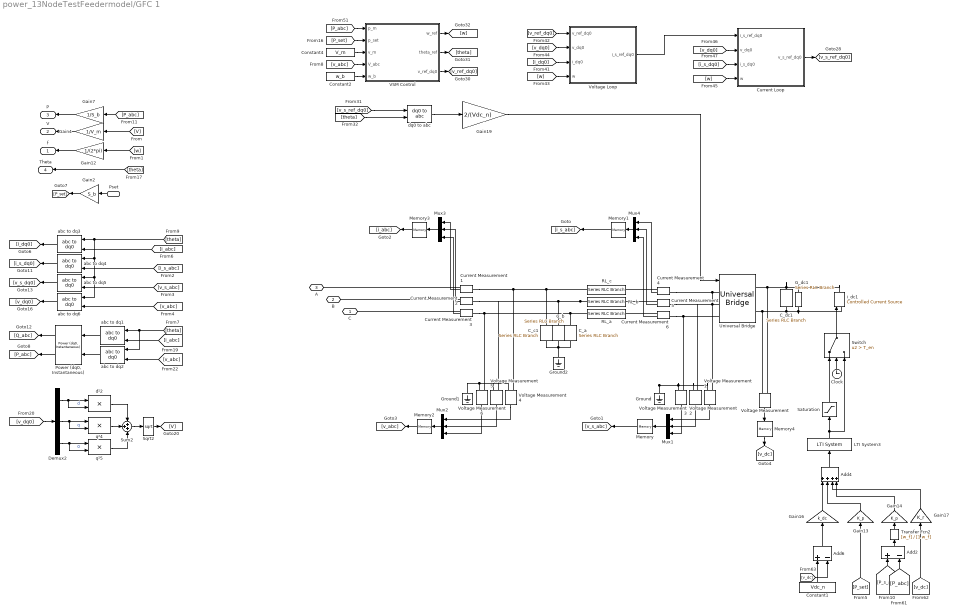
== system power_13NodeTestFeedermodel/GFC 1 ==
  Pset : Inport
  Add2 : Sum  Inputs=+-
  Add4 : Sum  Inputs=++++
  Add6 : Sum  Inputs=+-
  C_a : spsSeriesRLCBranchLib/Series RLC Branch  LConnTagsString=__new0  RConnTagsString=__new0  BranchType=C  Resistance=1  Inductance=1e-3  SetiL0=off  InitialCurrent=0  Capacitance=C_f  Setx0=off  InitialVoltage=165  Measurements=None
  C_b : spsSeriesRLCBranchLib/Series RLC Branch  LConnTagsString=__new0  RConnTagsString=__new0  BranchType=C  Resistance=1  Inductance=1e-3  SetiL0=off  InitialCurrent=0  Capacitance=C_f  Setx0=off  InitialVoltage=165  Measurements=None
  C_c1 : spsSeriesRLCBranchLib/Series RLC Branch  LConnTagsString=__new0  RConnTagsString=__new0  BranchType=C  Resistance=1  Inductance=1e-3  SetiL0=off  InitialCurrent=0  Capacitance=C_f  Setx0=off  InitialVoltage=165  Measurements=None
  C_dc1 : spsSeriesRLCBranchLib/Series RLC Branch  LConnTagsString=__new0  RConnTagsString=__new0  BranchType=C  Resistance=1  Inductance=1e-3  SetiL0=off  InitialCurrent=0  Capacitance=C_dc  Setx0=off  InitialVoltage=Vdc_n  Measurements=None
  Clock : Clock
  Constant1 : Constant  Value=Vdc_n
  Constant2 : Constant  Value=w_b
  Constant4 : Constant  Value=V_m
  Current Loop : Subsystem
  Current Measurement{1..6} (6 alike) : spsCurrentMeasurementLib/Current Measurement  PhasorSimulation=off  OutputType=Complex  PSBequivalent=0
  Demux2 : Demux  Outputs=3
  G_dc1 : spsSeriesRLCBranchLib/Series RLC Branch  LConnTagsString=__new0  RConnTagsString=__new0  BranchType=R  Resistance=R_dc  Inductance=1e-3  SetiL0=off  InitialCurrent=0  Capacitance=1e-6  Setx0=off  InitialVoltage=0  Measurements=None
  Gain12 : Gain  Gain=1/(2*pi)
  Gain13 : Gain  Gain=K_p
  Gain14 : Gain  Gain=K_p
  Gain16 : Gain  Gain=k_dc
  Gain17 : Gain  Gain=K_r
  Gain19 : Gain  Gain=2/(Vdc_n)
  Gain2 : Gain  Gain=S_b
  Gain4 : Gain  Gain=1/V_m
  Gain7 : Gain  Gain=1/S_b
  Ground : spsGroundLib/Ground  LConnTagsString=a
  Ground1 : spsGroundLib/Ground  LConnTagsString=a
  Ground2 : spsGroundLib/Ground  LConnTagsString=a
  LTI System3 : cstblocks/LTI System  sys=tf(1,[tau_dc 1])  IC=[]
  Memory{,1..4} (5 alike) : Memory
  Mux{1..4} (4 alike) : Mux  Inputs=3
  "Power (dq0, Instantaneous)" : spsPowerdq0InstantaneousLib/Power (dq0, Instantaneous)
      settings: SourceProductBaseCode=PS
  RL_a : spsSeriesRLCBranchLib/Series RLC Branch  LConnTagsString=__new0  RConnTagsString=__new0  BranchType=RL  Resistance=R_f  Inductance=L_f  SetiL0=off  InitialCurrent=0  Capacitance=1e-6  Setx0=off  InitialVoltage=0  Measurements=Branch voltage and current
  RL_b : spsSeriesRLCBranchLib/Series RLC Branch  LConnTagsString=__new0  RConnTagsString=__new0  BranchType=RL  Resistance=R_f  Inductance=L_f  SetiL0=off  InitialCurrent=0  Capacitance=1e-6  Setx0=off  InitialVoltage=0  Measurements=None
  RL_c : spsSeriesRLCBranchLib/Series RLC Branch  LConnTagsString=__new0  RConnTagsString=__new0  BranchType=RL  Resistance=R_f  Inductance=L_f  SetiL0=off  InitialCurrent=0  Capacitance=1e-6  Setx0=off  InitialVoltage=0  Measurements=None
  Saturation : Saturate  UpperLimit=i_ul  LowerLimit=i_ll
  Sqrt2 : Sqrt  SaturateOnIntegerOverflow=on
  Sum2 : Sum  Inputs=+++  InputSameDT=on  SaturateOnIntegerOverflow=on  OutDataTypeStr=Inherit: Same as first input
  Switch : Switch  Criteria=u2 > Threshold  Threshold=T_en
  Transfer Fcn2 : TransferFcn  Numerator=[w_f]  Denominator=[1 w_f]
  Universal Bridge : spsUniversalBridgeLib/Universal Bridge  Arms=3  SnubberResistance=1e5  SnubberCapacitance=inf  Device=Average-model based VSC  Ron=1e-3  Lon=0  ForwardVoltages="[  0  0  ]"  ForwardVoltage=0  GTOparameters=[ 10e-6 , 20e-6 ]  IGBTparameters=[ 1e-6 , 2e-6 ]  Measurements=None  Measurements_2=None  converterType=Rectifier
  VSM Control : Subsystem
  Voltage Loop : Subsystem
  Voltage Measurement{,1..6} (7 alike) : spsVoltageMeasurementLib/Voltage Measurement  PhasorSimulation=off  OutputType=Complex  PSBequivalent=0
  abc to dq{1..6} (6 alike) : spsabctodq0Lib/abc to dq0  Alignment=90 degrees behind phase A axis
  dq0 to abc : spsdq0toabcLib/dq0 to abc  Alignment=90 degrees behind phase A axis
  d²2 : Product  InputSameDT=on  RndMeth=Zero  SaturateOnIntegerOverflow=on  OutDataTypeStr=Inherit: Same as first input
  i_dc1 : spsControlledCurrentSourceLib/Controlled Current Source  Initialize=off  Source_Type=DC  Amplitude=i_dc  Phase=0  Frequency=0  Measurements=None
  q²4 : Product  InputSameDT=on  RndMeth=Zero  SaturateOnIntegerOverflow=on  OutDataTypeStr=Inherit: Same as first input
  q²5 : Product  InputSameDT=on  RndMeth=Zero  SaturateOnIntegerOverflow=on  OutDataTypeStr=Inherit: Same as first input
  C : PMIOPort  Side=Right
  B : PMIOPort  Port=2  Side=Right
  A : PMIOPort  Port=3  Side=Right
  f : Outport  VectorParamsAs1DForOutWhenUnconnected=off
  V : Outport  Port=2  VectorParamsAs1DForOutWhenUnconnected=off
  P : Outport  Port=3  VectorParamsAs1DForOutWhenUnconnected=off
  Theta : Outport  Port=4  VectorParamsAs1DForOutWhenUnconnected=off
  wires:
  Add4/1 -> LTI System3/1
  Clock/1 -> Switch/2
  Saturation/1 -> Switch/1
  LTI System3/1 -> Switch/3, Saturation/1
  Gain7/1 -> P/1
  [P_abc] -> Gain7/1
  Current Measurement6/1 -> Mux4/3
  Current Measurement5/1 -> Mux4/2
  Current Measurement4/1 -> Mux4/1
  Current Measurement3/1 -> Mux3/3
  Current Measurement2/1 -> Mux3/2
  Current Measurement1/1 -> Mux3/1
  Voltage Measurement4/1 -> Mux2/1
  Voltage Measurement5/1 -> Mux2/2
  Voltage Measurement6/1 -> Mux2/3
  Voltage Measurement3/1 -> Mux1/3
  Voltage Measurement2/1 -> Mux1/2
  Voltage Measurement1/1 -> Mux1/1
  [V] -> Gain4/1
  Gain2/1 -> [P_set]
  Pset/1 -> Gain2/1
  Gain12/1 -> f/1
  [w] -> Gain12/1
  Mux2/1 -> Memory2/1
  Mux3/1 -> Memory3/1
  Mux1/1 -> Memory/1
  abc to dq1/1 -> "Power (dq0, Instantaneous)"/2
  abc to dq2/1 -> "Power (dq0, Instantaneous)"/1
  [theta] -> abc to dq2/2, abc to dq1/2
  [v_abc] -> abc to dq2/1
  "Power (dq0, Instantaneous)"/2 -> [Q_abc]
  "Power (dq0, Instantaneous)"/1 -> [P_abc]
  [i_abc] -> abc to dq1/1
  Gain4/1 -> V/1
  [theta] -> Theta/1
  [i_abc] -> abc to dq3/1
  [i_s_abc] -> abc to dq4/1
  [v_abc] -> abc to dq6/1
  [v_s_abc] -> abc to dq5/1
  [theta] -> abc to dq4/2, abc to dq5/2, abc to dq6/2, abc to dq3/2
  abc to dq3/1 -> [i_dq0]
  abc to dq4/1 -> [i_s_dq0]
  abc to dq5/1 -> [v_s_dq0]
  abc to dq6/1 -> [v_dq0]
  [theta] -> dq0 to abc/2
  q²4/1 -> Sum2/2
  [v_dq0] -> Demux2/1
  q²5/1 -> Sum2/3
  Sum2/1 -> Sqrt2/1
  Demux2/3 -> q²5/1, q²5/2  "0"
  d²2/1 -> Sum2/1
  Demux2/2 -> q²4/1, q²4/2  "q"
  Demux2/1 -> d²2/1, d²2/2  "d"
  Sqrt2/1 -> [V]
  Mux4/1 -> Memory1/1
  Memory2/1 -> [v_abc]
  Memory3/1 -> [i_abc]
  Voltage Measurement/1 -> Memory4/1
  Memory4/1 -> [v_dc]
  Memory/1 -> [v_s_abc]
  Memory1/1 -> [i_s_abc]
  dq0 to abc/1 -> Gain19/1
  [w] -> Current Loop/4(w)
  [v_ref_dq0] -> Voltage Loop/1(v_ref_dq0)
  [i_dq0] -> Voltage Loop/3(i_dq0)
  Voltage Loop/1(i_s_ref_dq0) -> Current Loop/1(i_s_ref_dq0)
  [v_dq0] -> Current Loop/2(v_dq0)
  [i_s_dq0] -> Current Loop/3(i_s_dq0)
  Current Loop/1(v_s_ref_dq0) -> [v_s_ref_dq0]
  [w] -> Voltage Loop/4(w)
  [v_dq0] -> Voltage Loop/2(v_dq0)
  Switch/1 -> i_dc1/1
  Gain19/1 -> Universal Bridge/1
  [v_s_ref_dq0] -> dq0 to abc/1
  VSM Control/2(theta_ref) -> [theta]
  VSM Control/3(v_ref_dq0) -> [v_ref_dq0]
  Constant2/1 -> VSM Control/5(w_b)
  [P_set] -> VSM Control/2(p_set)
  [v_abc] -> VSM Control/4(V_abc)
  [P_abc] -> VSM Control/1(p_m)
  VSM Control/1(w_ref) -> [w]
  Constant4/1 -> VSM Control/3(v_m)
  [P_abc] -> Add2/2
  Gain14/1 -> Add4/4
  [P_set] -> Gain13/1
  Gain13/1 -> Add4/2
  Gain16/1 -> Add4/1
  Constant1/1 -> Add6/1
  Gain17/1 -> Add4/3
  Add2/1 -> Transfer Fcn2/1
  Transfer Fcn2/1 -> Gain14/1
  [v_dc] -> Add6/2
  Add6/1 -> Gain16/1
  [P_s_abc] -> Add2/1
  [v_dc] -> Gain17/1
  connections:
  RL_b/RConn1 -- Voltage Measurement5/LConn1 -- Current Measurement2/LConn1 -- C_b/LConn1
  Voltage Measurement6/LConn1 -- Current Measurement3/LConn1 -- C_a/LConn1 -- RL_a/RConn1
  Current Measurement4/RConn1 -- RL_c/LConn1
  Current Measurement6/RConn1 -- RL_a/LConn1
  Current Measurement5/RConn1 -- RL_b/LConn1
  Voltage Measurement/LConn1 -- Universal Bridge/RConn1 -- C_dc1/LConn1 -- G_dc1/LConn1 -- i_dc1/RConn1
  Voltage Measurement6/LConn2 -- Voltage Measurement5/LConn2 -- Voltage Measurement4/LConn2 -- Ground1/LConn1
  Ground/LConn1 -- Voltage Measurement2/LConn2 -- Voltage Measurement1/LConn2 -- Voltage Measurement3/LConn2
  Current Measurement3/RConn1 -- C/RConn1
  Current Measurement2/RConn1 -- B/RConn1
  Current Measurement1/RConn1 -- A/RConn1
  Current Measurement6/LConn1 -- Universal Bridge/LConn3 -- Voltage Measurement3/LConn1
  Universal Bridge/LConn2 -- Current Measurement5/LConn1 -- Voltage Measurement2/LConn1
  Universal Bridge/LConn1 -- Current Measurement4/LConn1 -- Voltage Measurement1/LConn1
  Universal Bridge/RConn2 -- Voltage Measurement/LConn2 -- C_dc1/RConn1 -- G_dc1/RConn1 -- i_dc1/LConn1
  C_b/RConn1 -- C_a/RConn1 -- Ground2/LConn1 -- C_c1/RConn1
  Voltage Measurement4/LConn1 -- Current Measurement1/LConn1 -- C_c1/LConn1 -- RL_c/RConn1

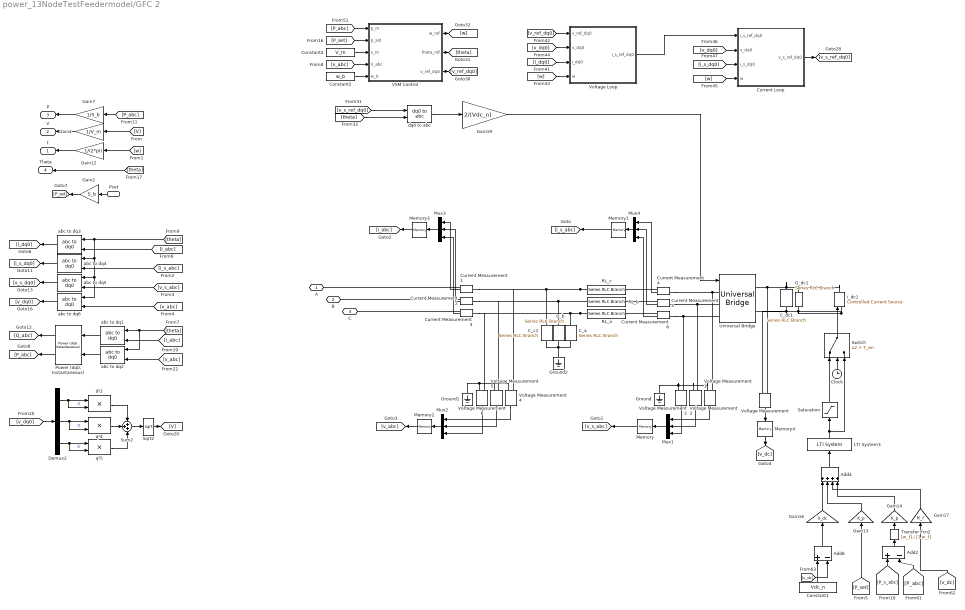
== system power_13NodeTestFeedermodel/GFC 2 ==
  Pset : Inport
  Add2 : Sum  Inputs=+-
  Add4 : Sum  Inputs=++++
  Add6 : Sum  Inputs=+-
  C_a : spsSeriesRLCBranchLib/Series RLC Branch  LConnTagsString=__new0  RConnTagsString=__new0  BranchType=C  Resistance=1  Inductance=1e-3  SetiL0=off  InitialCurrent=0  Capacitance=C_f  Setx0=off  InitialVoltage=165  Measurements=None
  C_b : spsSeriesRLCBranchLib/Series RLC Branch  LConnTagsString=__new0  RConnTagsString=__new0  BranchType=C  Resistance=1  Inductance=1e-3  SetiL0=off  InitialCurrent=0  Capacitance=C_f  Setx0=off  InitialVoltage=165  Measurements=None
  C_c1 : spsSeriesRLCBranchLib/Series RLC Branch  LConnTagsString=__new0  RConnTagsString=__new0  BranchType=C  Resistance=1  Inductance=1e-3  SetiL0=off  InitialCurrent=0  Capacitance=C_f  Setx0=off  InitialVoltage=165  Measurements=None
  C_dc1 : spsSeriesRLCBranchLib/Series RLC Branch  LConnTagsString=__new0  RConnTagsString=__new0  BranchType=C  Resistance=1  Inductance=1e-3  SetiL0=off  InitialCurrent=0  Capacitance=C_dc  Setx0=off  InitialVoltage=Vdc_n  Measurements=None
  Clock : Clock
  Constant1 : Constant  Value=Vdc_n
  Constant2 : Constant  Value=w_b
  Constant4 : Constant  Value=V_m
  Current Loop : Subsystem
  Current Measurement{1..6} (6 alike) : spsCurrentMeasurementLib/Current Measurement  PhasorSimulation=off  OutputType=Complex  PSBequivalent=0
  Demux2 : Demux  Outputs=3
  G_dc1 : spsSeriesRLCBranchLib/Series RLC Branch  LConnTagsString=__new0  RConnTagsString=__new0  BranchType=R  Resistance=R_dc  Inductance=1e-3  SetiL0=off  InitialCurrent=0  Capacitance=1e-6  Setx0=off  InitialVoltage=0  Measurements=None
  Gain12 : Gain  Gain=1/(2*pi)
  Gain13 : Gain  Gain=K_p
  Gain14 : Gain  Gain=K_p
  Gain16 : Gain  Gain=k_dc
  Gain17 : Gain  Gain=K_r
  Gain19 : Gain  Gain=2/(Vdc_n)
  Gain2 : Gain  Gain=S_b
  Gain4 : Gain  Gain=1/V_m
  Gain7 : Gain  Gain=1/S_b
  Ground : spsGroundLib/Ground  LConnTagsString=a
  Ground1 : spsGroundLib/Ground  LConnTagsString=a
  Ground2 : spsGroundLib/Ground  LConnTagsString=a
  LTI System3 : cstblocks/LTI System  sys=tf(1,[tau_dc 1])  IC=[]
  Memory{,1..4} (5 alike) : Memory
  Mux{1..4} (4 alike) : Mux  Inputs=3
  "Power (dq0, Instantaneous)" : spsPowerdq0InstantaneousLib/Power (dq0, Instantaneous)
      settings: SourceProductBaseCode=PS
  RL_a : spsSeriesRLCBranchLib/Series RLC Branch  LConnTagsString=__new0  RConnTagsString=__new0  BranchType=RL  Resistance=R_f  Inductance=L_f  SetiL0=off  InitialCurrent=0  Capacitance=1e-6  Setx0=off  InitialVoltage=0  Measurements=Branch voltage and current
  RL_b : spsSeriesRLCBranchLib/Series RLC Branch  LConnTagsString=__new0  RConnTagsString=__new0  BranchType=RL  Resistance=R_f  Inductance=L_f  SetiL0=off  InitialCurrent=0  Capacitance=1e-6  Setx0=off  InitialVoltage=0  Measurements=None
  RL_c : spsSeriesRLCBranchLib/Series RLC Branch  LConnTagsString=__new0  RConnTagsString=__new0  BranchType=RL  Resistance=R_f  Inductance=L_f  SetiL0=off  InitialCurrent=0  Capacitance=1e-6  Setx0=off  InitialVoltage=0  Measurements=None
  Saturation : Saturate  UpperLimit=i_ul  LowerLimit=i_ll
  Sqrt2 : Sqrt  SaturateOnIntegerOverflow=on
  Sum2 : Sum  Inputs=+++  InputSameDT=on  SaturateOnIntegerOverflow=on  OutDataTypeStr=Inherit: Same as first input
  Switch : Switch  Criteria=u2 > Threshold  Threshold=T_en
  Transfer Fcn2 : TransferFcn  Numerator=[w_f]  Denominator=[1 w_f]
  Universal Bridge : spsUniversalBridgeLib/Universal Bridge  Arms=3  SnubberResistance=1e5  SnubberCapacitance=inf  Device=Average-model based VSC  Ron=1e-3  Lon=0  ForwardVoltages="[  0  0  ]"  ForwardVoltage=0  GTOparameters=[ 10e-6 , 20e-6 ]  IGBTparameters=[ 1e-6 , 2e-6 ]  Measurements=None  Measurements_2=None  converterType=Rectifier
  VSM Control : Subsystem
  Voltage Loop : Subsystem
  Voltage Measurement{,1..6} (7 alike) : spsVoltageMeasurementLib/Voltage Measurement  PhasorSimulation=off  OutputType=Complex  PSBequivalent=0
  abc to dq{1..6} (6 alike) : spsabctodq0Lib/abc to dq0  Alignment=90 degrees behind phase A axis
  dq0 to abc : spsdq0toabcLib/dq0 to abc  Alignment=90 degrees behind phase A axis
  d²2 : Product  InputSameDT=on  RndMeth=Zero  SaturateOnIntegerOverflow=on  OutDataTypeStr=Inherit: Same as first input
  i_dc1 : spsControlledCurrentSourceLib/Controlled Current Source  Initialize=off  Source_Type=DC  Amplitude=i_dc  Phase=0  Frequency=0  Measurements=None
  q²4 : Product  InputSameDT=on  RndMeth=Zero  SaturateOnIntegerOverflow=on  OutDataTypeStr=Inherit: Same as first input
  q²5 : Product  InputSameDT=on  RndMeth=Zero  SaturateOnIntegerOverflow=on  OutDataTypeStr=Inherit: Same as first input
  A : PMIOPort  Side=Right
  B : PMIOPort  Port=2  Side=Right
  C : PMIOPort  Port=3  Side=Right
  f : Outport  VectorParamsAs1DForOutWhenUnconnected=off
  V : Outport  Port=2  VectorParamsAs1DForOutWhenUnconnected=off
  P : Outport  Port=3  VectorParamsAs1DForOutWhenUnconnected=off
  Theta : Outport  Port=4  VectorParamsAs1DForOutWhenUnconnected=off
  wires:
  [v_dc] -> Gain17/1
  [P_s_abc] -> Add2/1
  Add6/1 -> Gain16/1
  [v_dc] -> Add6/2
  Transfer Fcn2/1 -> Gain14/1
  Add2/1 -> Transfer Fcn2/1
  Gain17/1 -> Add4/3
  Constant1/1 -> Add6/1
  Gain16/1 -> Add4/1
  Gain13/1 -> Add4/2
  [P_set] -> Gain13/1
  Gain14/1 -> Add4/4
  [P_abc] -> Add2/2
  Constant4/1 -> VSM Control/3(v_m)
  VSM Control/1(w_ref) -> [w]
  [P_abc] -> VSM Control/1(p_m)
  [v_abc] -> VSM Control/4(V_abc)
  [P_set] -> VSM Control/2(p_set)
  Constant2/1 -> VSM Control/5(w_b)
  VSM Control/3(v_ref_dq0) -> [v_ref_dq0]
  VSM Control/2(theta_ref) -> [theta]
  [v_s_ref_dq0] -> dq0 to abc/1
  Gain19/1 -> Universal Bridge/1
  Switch/1 -> i_dc1/1
  [v_dq0] -> Voltage Loop/2(v_dq0)
  [w] -> Voltage Loop/4(w)
  Current Loop/1(v_s_ref_dq0) -> [v_s_ref_dq0]
  [i_s_dq0] -> Current Loop/3(i_s_dq0)
  [v_dq0] -> Current Loop/2(v_dq0)
  Voltage Loop/1(i_s_ref_dq0) -> Current Loop/1(i_s_ref_dq0)
  [i_dq0] -> Voltage Loop/3(i_dq0)
  [v_ref_dq0] -> Voltage Loop/1(v_ref_dq0)
  [w] -> Current Loop/4(w)
  dq0 to abc/1 -> Gain19/1
  Memory1/1 -> [i_s_abc]
  Memory/1 -> [v_s_abc]
  Memory4/1 -> [v_dc]
  Voltage Measurement/1 -> Memory4/1
  Memory3/1 -> [i_abc]
  Memory2/1 -> [v_abc]
  Mux4/1 -> Memory1/1
  Sqrt2/1 -> [V]
  Demux2/1 -> d²2/2, d²2/1  "d"
  Demux2/2 -> q²4/2, q²4/1  "q"
  d²2/1 -> Sum2/1
  Demux2/3 -> q²5/2, q²5/1  "0"
  Sum2/1 -> Sqrt2/1
  q²5/1 -> Sum2/3
  [v_dq0] -> Demux2/1
  q²4/1 -> Sum2/2
  [theta] -> dq0 to abc/2
  abc to dq6/1 -> [v_dq0]
  abc to dq5/1 -> [v_s_dq0]
  abc to dq4/1 -> [i_s_dq0]
  abc to dq3/1 -> [i_dq0]
  [theta] -> abc to dq3/2, abc to dq6/2, abc to dq5/2, abc to dq4/2
  [v_s_abc] -> abc to dq5/1
  [v_abc] -> abc to dq6/1
  [i_s_abc] -> abc to dq4/1
  [i_abc] -> abc to dq3/1
  [theta] -> Theta/1
  Gain4/1 -> V/1
  [i_abc] -> abc to dq1/1
  "Power (dq0, Instantaneous)"/1 -> [P_abc]
  "Power (dq0, Instantaneous)"/2 -> [Q_abc]
  [v_abc] -> abc to dq2/1
  [theta] -> abc to dq1/2, abc to dq2/2
  abc to dq2/1 -> "Power (dq0, Instantaneous)"/1
  abc to dq1/1 -> "Power (dq0, Instantaneous)"/2
  Mux1/1 -> Memory/1
  Mux3/1 -> Memory3/1
  Mux2/1 -> Memory2/1
  [w] -> Gain12/1
  Gain12/1 -> f/1
  Pset/1 -> Gain2/1
  Gain2/1 -> [P_set]
  [V] -> Gain4/1
  Voltage Measurement1/1 -> Mux1/1
  Voltage Measurement2/1 -> Mux1/2
  Voltage Measurement3/1 -> Mux1/3
  Voltage Measurement6/1 -> Mux2/3
  Voltage Measurement5/1 -> Mux2/2
  Voltage Measurement4/1 -> Mux2/1
  Current Measurement1/1 -> Mux3/1
  Current Measurement2/1 -> Mux3/2
  Current Measurement3/1 -> Mux3/3
  Current Measurement4/1 -> Mux4/1
  Current Measurement5/1 -> Mux4/2
  Current Measurement6/1 -> Mux4/3
  [P_abc] -> Gain7/1
  Gain7/1 -> P/1
  LTI System3/1 -> Saturation/1, Switch/3
  Saturation/1 -> Switch/1
  Clock/1 -> Switch/2
  Add4/1 -> LTI System3/1
  connections:
  RL_c/RConn1 -- C_c1/LConn1 -- Current Measurement1/LConn1 -- Voltage Measurement4/LConn1
  C_c1/RConn1 -- Ground2/LConn1 -- C_a/RConn1 -- C_b/RConn1
  i_dc1/LConn1 -- G_dc1/RConn1 -- C_dc1/RConn1 -- Voltage Measurement/LConn2 -- Universal Bridge/RConn2
  Voltage Measurement1/LConn1 -- Current Measurement4/LConn1 -- Universal Bridge/LConn1
  Voltage Measurement2/LConn1 -- Current Measurement5/LConn1 -- Universal Bridge/LConn2
  Voltage Measurement3/LConn1 -- Universal Bridge/LConn3 -- Current Measurement6/LConn1
  Current Measurement1/RConn1 -- A/RConn1
  Current Measurement2/RConn1 -- B/RConn1
  Current Measurement3/RConn1 -- C/RConn1
  Voltage Measurement3/LConn2 -- Voltage Measurement1/LConn2 -- Voltage Measurement2/LConn2 -- Ground/LConn1
  Ground1/LConn1 -- Voltage Measurement4/LConn2 -- Voltage Measurement5/LConn2 -- Voltage Measurement6/LConn2
  i_dc1/RConn1 -- G_dc1/LConn1 -- C_dc1/LConn1 -- Universal Bridge/RConn1 -- Voltage Measurement/LConn1
  Current Measurement5/RConn1 -- RL_b/LConn1
  Current Measurement6/RConn1 -- RL_a/LConn1
  Current Measurement4/RConn1 -- RL_c/LConn1
  RL_a/RConn1 -- C_a/LConn1 -- Current Measurement3/LConn1 -- Voltage Measurement6/LConn1
  C_b/LConn1 -- Current Measurement2/LConn1 -- Voltage Measurement5/LConn1 -- RL_b/RConn1
